simulink model "Simu_2"  (R2013a)
settings: Solver=ode45  StartTime=0.0  StopTime=3  RelTol=1e-3
libraries: fl_lib x6, nesl_utility x3
settings Model: Creator=Polotto  LastModifiedBy=Polotto

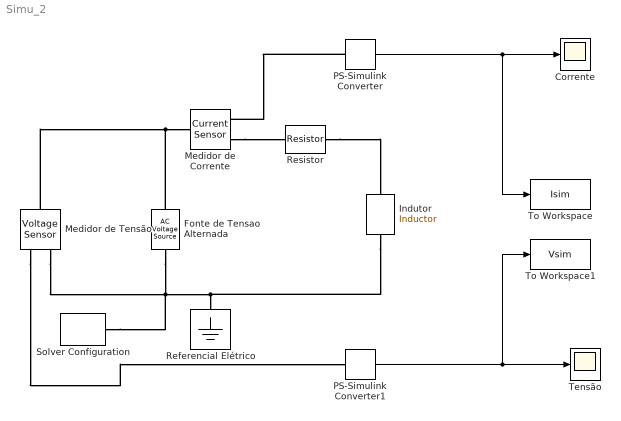
== system Simu_2 ==
  Corrente : Scope
      settings: YMin=-175  YMax=175
  Fonte de Tensao Alternada : fl_lib/Electrical/Electrical Sources/AC Voltage Source  amp=127*sqrt(2) V  shift=0 deg  frequency=60 Hz  omega=0 rad/s  i_Log=off  v_Log=off  LocalVarNames=|i|v  LocalVarDescs=|i|v  LocalVarLogging=[0 0]
  Indutor : fl_lib/Electrical/Electrical Elements/Inductor  l=10 mH  i0=0 A  r=0 Ohm  g=1e-9 1/Ohm  i_Log=off  v_Log=off  i_L_Log=off  LocalVarNames=|i|v|i_L  LocalVarDescs=|i|v|Internal variable for current through inductor term  LocalVarLogging=[0 0 0]
  Medidor de Corrente : fl_lib/Electrical/Electrical Sensors/Current Sensor  i1_Log=off  v1_Log=off  LocalVarNames=|i1|v1  LocalVarDescs=|i1|v1  LocalVarLogging=[0 0]
  Medidor de Tensão : fl_lib/Electrical/Electrical Sensors/Voltage Sensor  i1_Log=off  v1_Log=off  LocalVarNames=|i1|v1  LocalVarDescs=|i1|v1  LocalVarLogging=[0 0]
  PS-Simulink Converter : nesl_utility/PS-Simulink Converter  PhysicalDomain=network_engine_domain  SubClassName=ps_output  LeftPortType=input  RightPortType=output  PseudoPeriodic=off  Frequencies=[]  Unit=1  AffineConversion=off
  PS-Simulink Converter1 : nesl_utility/PS-Simulink Converter  PhysicalDomain=network_engine_domain  SubClassName=ps_output  LeftPortType=input  RightPortType=output  PseudoPeriodic=off  Frequencies=[]  Unit=1  AffineConversion=off
  Referencial Elétrico : fl_lib/Electrical/Electrical Elements/Electrical Reference  i_Log=off  LocalVarNames=|i  LocalVarDescs=|i  LocalVarLogging=0
  Resistor : fl_lib/Electrical/Electrical Elements/Resistor  R=10 Ohm  i_Log=off  v_Log=off  LocalVarNames=|i|v  LocalVarDescs=|i|v  LocalVarLogging=[0 0]
  Solver Configuration : nesl_utility/Solver Configuration  PhysicalDomain=network_engine_domain  SubClassName=solver  LeftPortType=input  RightPortType=generic  Accelerate=off  Tones=[]  Harmonics=[]  SimulateNoise=off  Profile=off  UseLocalSampling=off  EnableSwitchedLinearOptims=on  FrequencyDomain=off  UseCCode=off  UseNewInitialization=off  DoDC=off  ResidualTolerance=1e-09  UseLocalSolver=on  LocalSolverChoice=NE_BACKWARD_EULER_ADVANCER  LocalSolverSampleTime=0.0001  DoFixedCost=on  MaxNonlinIter=5  MaxModeIter=2  LinearAlgebra=Sparse  DelaysMemoryBudget=1024
  Tensão : Scope
      settings: YMin=-175  YMax=175
  To Workspace : ToWorkspace  VariableName=Isim  SampleTime=-1  SaveFormat=Structure With Time
  To Workspace1 : ToWorkspace  VariableName=Vsim  SampleTime=-1  SaveFormat=Structure With Time
  wires:
  PS-Simulink Converter/1 -> To Workspace/1, Corrente/1
  PS-Simulink Converter1/1 -> To Workspace1/1, Tensão/1
  connections:
  Fonte de Tensao Alternada/RConn1 -- Solver Configuration/RConn1 -- Indutor/RConn1 -- Referencial Elétrico/LConn1 -- Medidor de Tensão/RConn2
  Fonte de Tensao Alternada/LConn1 -- Medidor de Corrente/LConn1 -- Medidor de Tensão/LConn1
  Medidor de Corrente/RConn2 -- Resistor/LConn1
  PS-Simulink Converter/LConn1 -- Medidor de Corrente/RConn1
  Medidor de Tensão/RConn1 -- PS-Simulink Converter1/LConn1
  Resistor/RConn1 -- Indutor/LConn1
